simulink model "Day3_2"  (R2022b)
settings: Solver=FixedStepDiscrete  StartTime=0.0  StopTime=inf  FixedStep=0.01  RelTol=1e-3
libraries: statsLibrary x1
settings Model: Creator=user  LastModifiedBy=user
settings OptimizationCC: DefaultUnderspecifiedDataType=single
settings RTWCC: GenCodeOnly=on

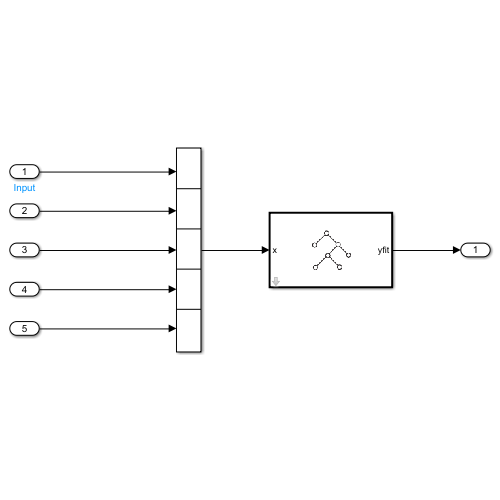
[thumbnail: Simulink's stored preview of the top-level diagram]
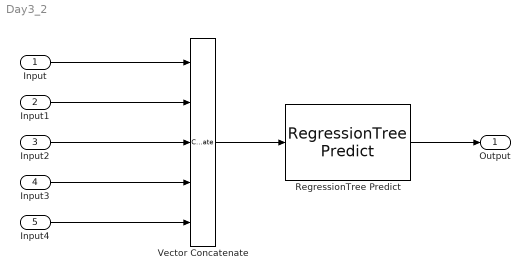
== system Day3_2 ==
  Input : Inport
  Input1 : Inport  Port=2
  Input2 : Inport  Port=3
  Input3 : Inport  Port=4
  Input4 : Inport  Port=5
  RegressionTree Predict : statsLibrary/Regression/RegressionTree Predict  TrainedLearner=trainedModel.RegressionTree  OutMin=[]  OutMax=[]
  Vector Concatenate : Concatenate  NumInputs=5
  Output : Outport
  wires:
  Input/1 -> Vector Concatenate/1
  Input1/1 -> Vector Concatenate/2
  Input2/1 -> Vector Concatenate/3
  Input3/1 -> Vector Concatenate/4
  Input4/1 -> Vector Concatenate/5
  Vector Concatenate/1 -> RegressionTree Predict/1
  RegressionTree Predict/1 -> Output/1
